simulink model "workingImpedance"  (R2018b)
settings: Solver=VariableStepAuto  StartTime=0.0  StopTime=50  RelTol=1e-3
libraries: simulink x1
settings Model: Creator=holyCow  LastModifiedBy=holyCow

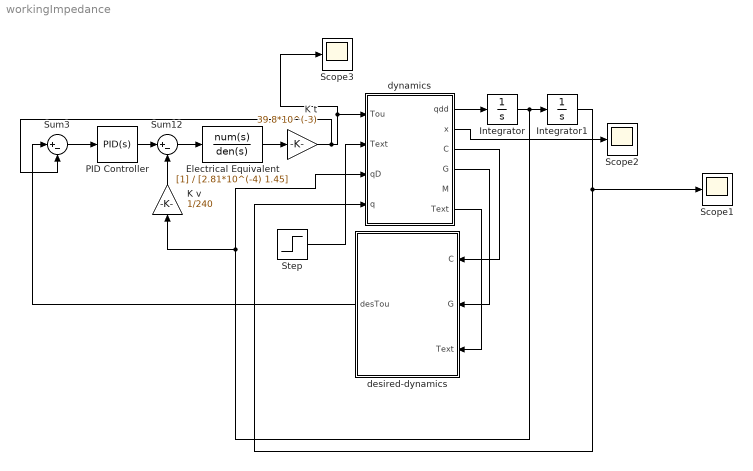
== system workingImpedance ==
  Electrical Equivalent : TransferFcn  Denominator=[2.81*10^(-4) 1.45]
  Integrator : Integrator
  Integrator1 : Integrator
  K t : Gain  Gain=39.8*10^(-3)
  K v : Gain  Gain=1/240
  PID Controller : simulink/Continuous/PID Controller  Controller=PID  Form=Parallel  TimeDomain=Continuous-time  SampleTime=-1  IntegratorMethod=Forward Euler  FilterMethod=Forward Euler  ControllerParametersSource=internal  P=1  I=1  D=0  UseFilter=on  N=100  TunerSelectOption=Transfer Function Based (PID Tuner App)  InitialConditionSource=internal  InitialConditionForIntegrator=0  InitialConditionForFilter=0  DifferentiatorICPrevScaledInput=0  ExternalReset=none  TrackingMode=off  Kt=1  LimitOutput=off  UpperSaturationLimit=inf  LowerSaturationLimit=-inf  LinearizeAsGain=on  AntiWindupMode=none  Kb=1  POutMin=[]  POutMax=[]  IOutMin=[]  IOutMax=[]  DOutMin=[]  DOutMax=[]  NOutMin=[]  NOutMax=[]  SumOutMin=[]  SumOutMax=[]  SaturationOutMin=[]  SaturationOutMax=[]  PParamMin=[]  PParamMax=[]  IParamMin=[]  IParamMax=[]  DParamMin=[]  DParamMax=[]  NParamMin=[]  NParamMax=[]  KbParamMin=[]  KbParamMax=[]  KtParamMin=[]  KtParamMax=[]  KbOutMin=[]  KbOutMax=[]  KtOutMin=[]  KtOutMax=[]  IntegratorOutMin=[]  IntegratorOutMax=[]  FilterOutMin=[]  FilterOutMax=[]  SumI1OutMin=[]  SumI1OutMax=[]  SumI2OutMin=[]  SumI2OutMax=[]  SumI3OutMin=[]  SumI3OutMax=[]  SumI4OutMin=[]  SumI4OutMax=[]  SumDOutMin=[]  SumDOutMax=[]  DifferentiatorOutMin=[]  DifferentiatorOutMax=[]  FilterDiffOutCoefMin=[]  FilterDiffOutCoefMax=[]  ReciprocalOutMin=[]  ReciprocalOutMax=[]  SumDenOutMin=[]  SumDenOutMax=[]  SumNumOutMin=[]  SumNumOutMax=[]  DivideOutMin=[]  DivideOutMax=[]  IntegratorContinuousStateAttributes=''  IntegratorStateMustResolveToSignalObject=off  IntegratorRTWStateStorageClass=Auto  FilterContinuousStateAttributes=''  FilterStateMustResolveToSignalObject=off  FilterRTWStateStorageClass=Auto  ParallelPVariant=InternalParameters  IdealPVariant=Disabled  IVariant=InternalParameters  DVariant=InternalParameters  IntegratorVariant=Continuous  SatVariant=Disabled  AWVariant=Passthrough  PCopyVariant=Disabled  TRVariant=Disabled  FdbkBlocksVariant=Forward  IdealPFdbkVariant=Disabled  SatFdbkVariant=Disabled  DerivativeFilterVariant=ContFilter  NVariant=InternalParameters  NCopyVariant=Disabled  FilterICVariant=InternalICsFilter  IntegratorICVariant=InternalICs  ExternalResetVariant=Disabled  TRSumVariant=Passthrough  SumFdbkVariant=Disabled  SumVariant=Sum_PID
  Scope1 : Scope
  Scope2 : Scope
  Scope3 : Scope
  Step : Step  Time=5  After=0  SampleTime=0
  Sum12 : Sum  Inputs=|+-
  Sum3 : Sum  Inputs=|+-
  desired-dynamics : MATLAB Function  TreatAsAtomicUnit=on
  dynamics : MATLAB Function  TreatAsAtomicUnit=on
  wires:
  Integrator1/1 -> Scope1/1, dynamics/4(q)
  Step/1 -> dynamics/2("Text ")
  desired-dynamics/1(desTou) -> Sum3/1
  Sum12/1 -> Electrical Equivalent/1
  dynamics/1(qdd) -> Integrator/1
  Integrator/1 -> K v/1, dynamics/3(qD), Integrator1/1
  PID Controller/1 -> Sum12/1
  Sum3/1 -> PID Controller/1
  dynamics/3(C) -> desired-dynamics/1(C)
  Electrical Equivalent/1 -> K t/1
  dynamics/2(x) -> Scope2/1
  dynamics/4(G) -> desired-dynamics/2(G)
  dynamics/6(Text) -> desired-dynamics/3(Text)
  K v/1 -> Sum12/2
  K t/1 -> Scope3/1, dynamics/1(Tou), Sum3/2

== matlab function workingImpedance/desired-dynamics ==
  data: C input; G input; Text input; desTou output
function desTou = fcn(C, G, Text)
%params;
Kb = 0.1;
Kk = 0.2;

desTou = Kb*C + Kk*G - Text;

== matlab function workingImpedance/dynamics ==
  data: Tou input; Text input; qD input; qdd output; q input; x output; C output; G output; M output; Text output
function [qdd, x, C, G, M, Text]= fcn(Tou, Text, qD, q)
l = 0.265;
m = 0.170;
a = 0.110;
b = 0.090;

g = 9.81;

m1 = 2.5;
m2 = 0.2;
mr = 0.1;
mf = 0.075;

% measure of radius
rr = 0.110/2;
rf = 0.075/2;

delta = rr - rf;

% l*sin(q2) + delta = m*sin(q1 - q2)
ta = (l/m + cos(q))^2 + (sin(q))^2;
tb = -2*(delta/m)*sin(q);
tc = (delta/m)^2 - (l/m + cos(q))^2;

q2 = acos((-tb + sqrt(tb^2 - 4*ta*tc))/(2*ta));
k = -1/(1 + ((l*cos(q2))/(m*cos(q - q2))));
%q2D = k * q1D;

x = sqrt(l^2 + m^2 - delta^2 + 2*l*m*cos(q));
c = ((-l*m*sin(q))/x);
%xD = c * q1D;

s = -1 * (l*k*m*sin(q2)*cos(q - q2) - l*m*cos(q2)*sin(q - q2)*(1 - k))/((l*cos(q2) + m*cos(q - q2))^2);
u = (l*m*(c*sin(q) - x*cos(q)))/(x^2);

%kD = s * q1D;
%cD = u * q1D;

%xa = a*cos(q2);
%xaD = -a*sin(q2)*q2D;

%ya = rr + a*sin(q2);
%yaD = a*cos(q2)*q2D;

%xb = x - b*cos(q - q2);
%xbD = xD + b*sin(q1 - q2)*(q1D - q2D);

%yb = rf + b*sin(q1 - q2);
%ybD = b*cos(q1 - q2)*(q1D - q2D);

%K = 0.5*m1*(xaD^2 + yaD^2) + 0.5*m2*(xbD^2 + ybD^2) + 0.75*mf*xD^2;
%P = mr*g*rr + mf*g*rf + m1*g*ya + m2*g*yb;

M = m1*(a^2)*(k^2) + (m2 + 1.5*mf)*(c^2) + m2*(b^2)*((1-k)^2) + 2*m2*b*sin(q - q2)*c*(1-k);

ctemp = cos(q - q2)*c*((1-k)^2) + sin(q - q2)*u*(1-k) - sin(q - q2)*c*s;
C = (m1*(a^2)*k*s + (m2 + 1.5*mf)*c*u - m2*(b^2)*s*(1-k) + m2*b*ctemp) * (qD^2);

G = m1*g*a*cos(q2)*k + m2*g*b*cos(q - q2)*(1 - k);

%N2 = (m1*g*xa + m2*g*xb)/(x);
%N1 = (((m1+m2)*x - m1*xa - m2*xb)*g)/(x);
%T_ext = Text + N1*l*cos(q2) - N2*m*cos(q1 - q2);
%Text = Fx*l*sin(q - q2) - Fy*m*cos(q - q2);
qdd = (Tou + Text - C - G)/M;
